simulink model "fixedEEControlR2016av2"  (Simulink 8.7)
settings: Solver=ode5  StartTime=0.0  StopTime=inf  FixedStep=0.01  RelTol=1e-3
libraries: WBToolboxLibrary x12
settings Model: Creator=yeshi  LastModifiedBy=yeshi
settings DataIOCC: LimitDataPoints=off  SaveFormat=Dataset
settings DebuggingCC: UnderspecifiedInitializationDetection=Simplified  MergeDetectMultiDrivingBlocksExec=error
settings HardwareCC: ProdBitPerPointer=64  ProdLargestAtomicFloat=Float  ProdIntDivRoundTo=Zero  ProdEndianess=LittleEndian  ProdWordSize=64  ProdHWDeviceType=Intel->x86-64 (Windows64)
settings ModelReferenceCC: PropagateSignalLabelsOutOfModel=on
settings ConfigComp: CovModelRefEnable=off

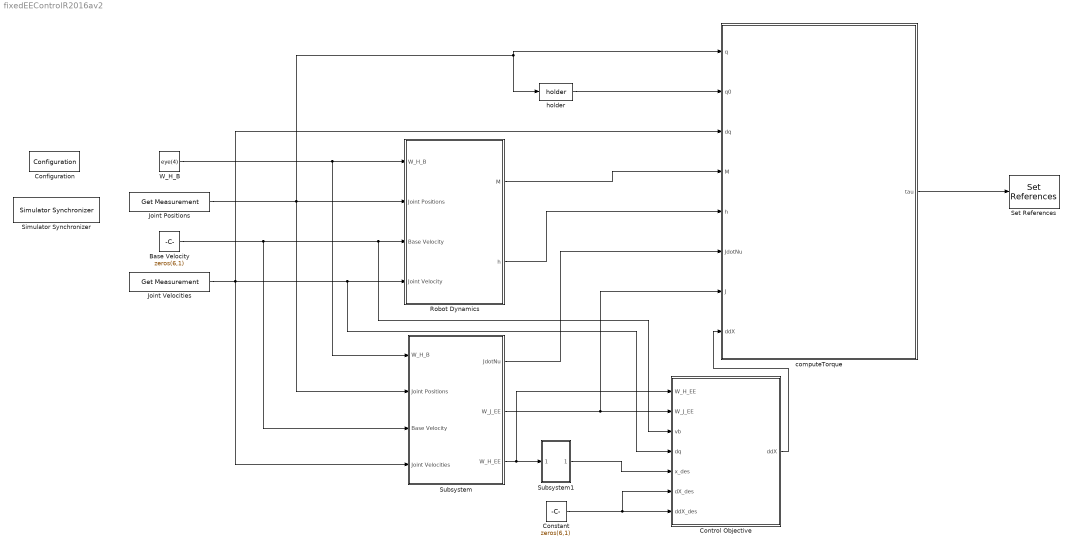
== system fixedEEControlR2016av2 ==
  Base Velocity : Constant  Value=zeros(6,1)
  Configuration : WBToolboxLibrary/Utilities/Configuration  ConfigSource=Workspace  ConfigObject='WBTConfigRobot'
  Constant : Constant  Value=zeros(6,1)
  Control Objective : MATLAB Function  TreatAsAtomicUnit=on
  Joint Positions : WBToolboxLibrary/wholeBodyStates/Get Measurement  measuredType=Joints Position
  Joint Velocities : WBToolboxLibrary/wholeBodyStates/Get Measurement  measuredType=Joints Velocity
  Robot Dynamics : Subsystem
  Set References : WBToolboxLibrary/wholeBodyActuators/Set References  controlType=Torque  refSpeed=50
  Simulator Synchronizer : WBToolboxLibrary/Utilities/Simulator Synchronizer  period=0.01  serverPortName='/clock/rpc'  clientPortName='/WBT_synchronizer/rpc:o'
  Subsystem : Subsystem
  Subsystem1 : Subsystem
  W_H_B : Constant  Value=eye(4)
  computeTorque : MATLAB Function  TreatAsAtomicUnit=on
  "holder " : WBToolboxLibrary/Utilities/holder 
  wires:
  W_H_B/1 -> Subsystem/1(W_H_B), Robot Dynamics/1(W_H_B)
  Joint Positions/1 -> "holder "/1, computeTorque/1(q), Subsystem/2(Joint Positions), Robot Dynamics/2(Joint Positions)
  Joint Velocities/1 -> computeTorque/3(dq), Subsystem/4(Joint Velocities), Control Objective/4(dq), Robot Dynamics/4(Joint Velocity)
  Robot Dynamics/1(M) -> computeTorque/4(M)
  Robot Dynamics/2(h) -> computeTorque/5(h)
  Subsystem/1(JdotNu) -> computeTorque/6(JdotNu)
  Subsystem/2(W_J_EE) -> Control Objective/2(W_J_EE), computeTorque/7(J)
  "holder "/1 -> computeTorque/2(q0)
  computeTorque/1(tau) -> Set References/1
  Subsystem/3(W_H_EE) -> Control Objective/1(W_H_EE), Subsystem1/1(In1)
  Subsystem1/1(Xdes) -> Control Objective/5(x_des)
  Constant/1 -> Control Objective/7(ddX_des), Control Objective/6(dX_des)
  Control Objective/1(ddX) -> computeTorque/8(ddX)
  Base Velocity/1 -> Subsystem/3(Base Velocity), Control Objective/3(vb), Robot Dynamics/3(Base Velocity)

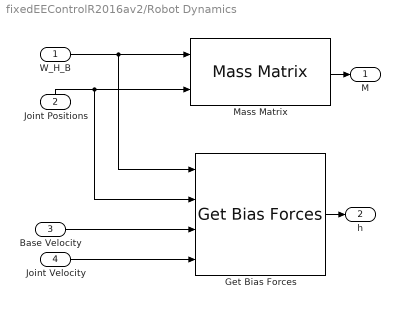
== system fixedEEControlR2016av2/Robot Dynamics ==
  W_H_B : Inport
  Joint Positions : Inport  Port=2
  Base Velocity : Inport  Port=3
  Joint Velocity : Inport  Port=4
  Get Bias Forces : WBToolboxLibrary/wholeBodyModel/Dynamics/Get Bias Forces
  Mass Matrix : WBToolboxLibrary/wholeBodyModel/Dynamics/Mass Matrix
  M : Outport
  h : Outport  Port=2
  wires:
  Base Velocity/1 -> Get Bias Forces/3
  Joint Velocity/1 -> Get Bias Forces/4
  Mass Matrix/1 -> M/1
  Get Bias Forces/1 -> h/1
  W_H_B/1 -> Get Bias Forces/1, Mass Matrix/1
  Joint Positions/1 -> Get Bias Forces/2, Mass Matrix/2

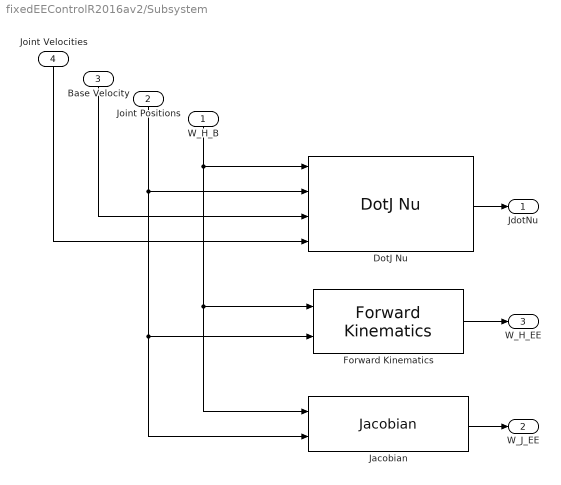
== system fixedEEControlR2016av2/Subsystem ==
  W_H_B : Inport
  Joint Positions : Inport  Port=2
  Base Velocity : Inport  Port=3
  Joint Velocities : Inport  Port=4
  DotJ Nu : WBToolboxLibrary/wholeBodyModel/Jacobians/DotJ Nu  frameName=CONFIG.EE
  Forward Kinematics : WBToolboxLibrary/wholeBodyModel/Kinematics/Forward Kinematics  frameName=CONFIG.EE
  Jacobian : WBToolboxLibrary/wholeBodyModel/Jacobians/Jacobian  frameName=CONFIG.EE
  JdotNu : Outport
  W_J_EE : Outport  Port=2
  W_H_EE : Outport  Port=3
  wires:
  Forward Kinematics/1 -> W_H_EE/1
  W_H_B/1 -> Jacobian/1, Forward Kinematics/1, DotJ Nu/1
  Joint Velocities/1 -> DotJ Nu/4
  Base Velocity/1 -> DotJ Nu/3
  DotJ Nu/1 -> JdotNu/1
  Jacobian/1 -> W_J_EE/1
  Joint Positions/1 -> Jacobian/2, Forward Kinematics/2, DotJ Nu/2

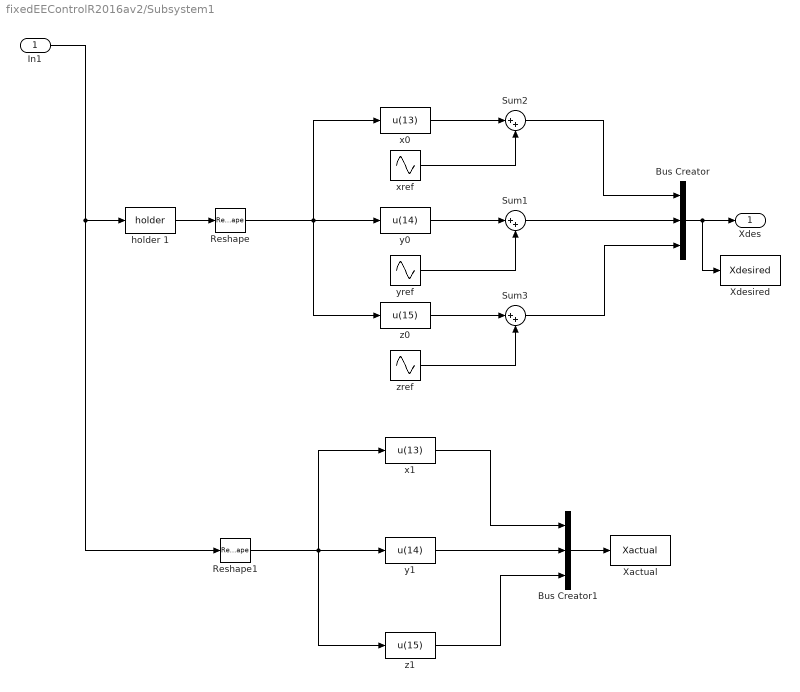
== system fixedEEControlR2016av2/Subsystem1 ==
  In1 : Inport
  Bus Creator : BusCreator  Inputs=3
  Bus Creator1 : BusCreator  Inputs=3
  Reshape : Reshape
  Reshape1 : Reshape
  Sum1 : Sum  Inputs=|++
  Sum2 : Sum  Inputs=|++
  Sum3 : Sum  Inputs=|++
  Xactual : ToWorkspace  VariableName=Xactual  SaveFormat=Timeseries  SampleTime=-1
  Xdesired : ToWorkspace  VariableName=Xdesired  SaveFormat=Timeseries  SampleTime=-1
  holder 1 : WBToolboxLibrary/Utilities/holder 
  x0 : Fcn  Expr=u(13)
  x1 : Fcn  Expr=u(13)
  xref : Sin  Amplitude=0  SampleTime=0
  y0 : Fcn  Expr=u(14)
  y1 : Fcn  Expr=u(14)
  yref : Sin  Amplitude=0.05  SampleTime=0
  z0 : Fcn  Expr=u(15)
  z1 : Fcn  Expr=u(15)
  zref : Sin  Amplitude=0.05  Phase=pi/2  SampleTime=0
  Xdes : Outport
  wires:
  Reshape1/1 -> y1/1, z1/1, x1/1
  Bus Creator1/1 -> Xactual/1
  z1/1 -> Bus Creator1/3
  y1/1 -> Bus Creator1/2
  In1/1 -> Reshape1/1, holder 1/1
  holder 1/1 -> Reshape/1
  Reshape/1 -> z0/1, y0/1, x0/1
  x0/1 -> Sum2/1
  xref/1 -> Sum2/2
  y0/1 -> Sum1/1
  yref/1 -> Sum1/2
  z0/1 -> Sum3/1
  Sum2/1 -> Bus Creator/1
  zref/1 -> Sum3/2
  Sum1/1 -> Bus Creator/2
  Sum3/1 -> Bus Creator/3
  Bus Creator/1 -> Xdes/1, Xdesired/1
  x1/1 -> Bus Creator1/1

== matlab function Control Objective ==
  data: W_H_EE input double; ddX output double; W_J_EE input double; vb input double; dq input double; x_des input double; dX_des input double; ddX_des input double
function ddX = controlObjective(W_H_EE,W_J_EE,vb,dq,x_des,dX_des,ddX_des)
   
    x = W_H_EE(1:3,4)-x_des;
    X = [x' 0 0 0]';
    
    nu = [vb' dq']';
    dX = W_J_EE*nu-dX_des;
   
    kp = 200;
    kd = 2*sqrt(kp);

    ddX = ddX_des-kp*X-kd*dX; 

end

== matlab function computeTorque ==
  data: q input double; tau output double; q0 input double; dq input double; M input double; h input double; JdotNu input double; J input double; ddX input double
function tau = computeTorque(q,q0,dq,M,h,JdotNu,J,ddX)

    dofs = 11;
    S = [zeros(dofs,6) eye(dofs)]';
    
    epsilon = 1e-20;
    lambda = J*inv(M)*S;
    alpha  = pinvDamped(lambda,epsilon);
    
    tau_pri = alpha*(ddX + J*inv(M)*h - JdotNu);
    
    nullspace = eye(size(lambda,2))- alpha*lambda;
    kp = 10;
    kd = 5;%2*sqrt(kp);
    tau_null = pinvDamped(S,epsilon)*h - kp*(q-q0) - kd*dq;
    
    tau = tau_pri + nullspace*tau_null;

end
